simulink model "model5"  (R2022a)
settings: Solver=VariableStepAuto  StartTime=0.0  StopTime=20  RelTol=1e-3
values from neighbouring files (symbols this model uses):
  A = [0 0 0 1 0 0; 0 0 0 0 1 0; 0 0 0 0 0 1; 0 6.5 -10 -alpha 0 0; a_51 a_52 a_53 a_54 a_55 a_56; 5 -3.6 0 0 0 -gamma]    [ME5401.m]
  B = [0 0; 0 0; 0 0; beta 11.2; b_51 b_52; 40 delta]    [ME5401.m]    (also in unity_place.m = B*q)
  C = [1 0 0 0 0 0; 0 1 0 0 0 0; 0 0 1 0 0 0]    [ME5401.m]    (also in place_pole.m = CC; unity_place.m = W_c)
  K_5 = real(my_lqr(A_5, B_5, Q, R))    [ME5401.m]
  L = place_pole(A',C',[-5 -10 -15 -20 -25 -30])'    [ME5401.m]
  Y_sp = -0.1*C*A^(-1)*B*[-0.5 + (a-b)/20; 0.1+(b-c)/(a+d+10)]    [ME5401.m]
settings Model: Creator=jiaya  LastModifiedBy=jiaya
settings ModelReferenceCC: EnableRefExpFcnMdlSchedulingChecks=off
settings RTWCC: Description=Generic Real-Time Target

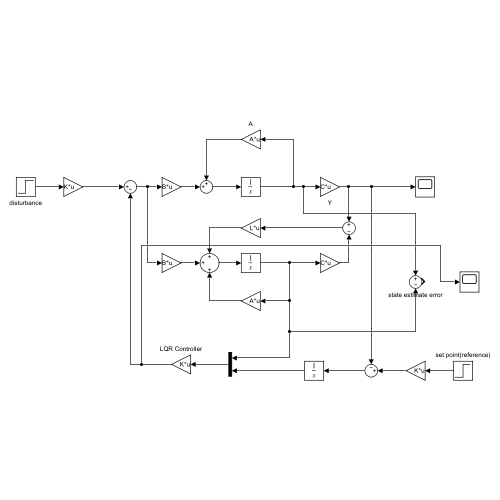
[thumbnail: Simulink's stored preview of the top-level diagram]
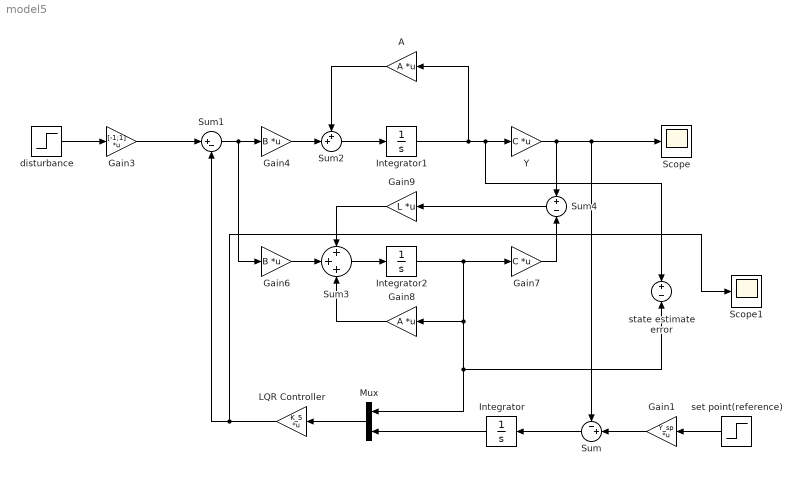
== system model5 ==
  A : Gain  Gain=A  Multiplication=Matrix(K*u)
  Gain1 : Gain  Gain=Y_sp  Multiplication=Matrix(K*u)
  Gain3 : Gain  Gain=[-1;1]  Multiplication=Matrix(K*u)
  Gain4 : Gain  Gain=B  Multiplication=Matrix(K*u)
  Gain6 : Gain  Gain=B  Multiplication=Matrix(K*u)
  Gain7 : Gain  Gain=C  Multiplication=Matrix(K*u)
  Gain8 : Gain  Gain=A  Multiplication=Matrix(K*u)
  Gain9 : Gain  Gain=L  Multiplication=Matrix(K*u)
  Integrator : Integrator
  Integrator1 : Integrator
  Integrator2 : Integrator
  LQR Controller : Gain  Gain=K_5  Multiplication=Matrix(K*u)
  Mux : Mux  Inputs=2
  Scope : Scope
  Scope1 : Scope
  Sum : Sum  Inputs=-+|
  Sum1 : Sum  Inputs=|+-
  Sum2 : Sum  Inputs=++|
  Sum3 : Sum  Inputs=+++
  Sum4 : Sum  Inputs=+|-
  Y : Gain  Gain=C  Multiplication=Matrix(K*u)
  disturbance : Step  Time=10  SampleTime=0
  set point(reference) : Step  Time=0  SampleTime=0
  state estimate error : Sum  Inputs=+-
  wires:
  Y/1 -> Sum4/1, Scope/1, Sum/1
  Gain1/1 -> Sum/2
  set point(reference)/1 -> Gain1/1
  Sum/1 -> Integrator/1
  Integrator/1 -> Mux/2
  Mux/1 -> LQR Controller/1
  LQR Controller/1 -> Scope1/1, Sum1/2
  Gain3/1 -> Sum1/1
  disturbance/1 -> Gain3/1
  Integrator1/1 -> A/1, state estimate error/1, Y/1
  Sum2/1 -> Integrator1/1
  Sum1/1 -> Gain6/1, Gain4/1
  A/1 -> Sum2/1
  Gain4/1 -> Sum2/2
  Sum3/1 -> Integrator2/1
  Integrator2/1 -> state estimate error/2, Mux/1, Gain8/1, Gain7/1
  Gain7/1 -> Sum4/2
  Sum4/1 -> Gain9/1
  Gain8/1 -> Sum3/3
  Gain6/1 -> Sum3/2
  Gain9/1 -> Sum3/1
